simulink model "helicoptertemplate_mp_v2c"  (R2021b)
settings: Solver=ode45  StartTime=0.0  StopTime=Tsim  RelTol=1e-3
InitFcn:
  | hwinit
values from neighbouring files (symbols this model uses):
  A = sysd.A    [MPC_Reference_track.m]    (also in MPC_Reference_track_offset.m; MPC_init_v2.m; MPC_init_v3.m; modelDynamics.m = [0, 1; -(1/J)*g*Mcw*L1*cos(-0.38), -(1/J)*C_alpha])
  B = sysd.B    [MPC_Reference_track.m]    (also in MPC_Reference_track_offset.m; MPC_init_v2.m; MPC_init_v3.m; modelDynamics.m = [0; (1/J)*L2])
  C = sysd.C    [MPC_Reference_track.m]    (also in MPC_Reference_track_offset.m; MPC_init_v2.m; MPC_init_v3.m; modelDynamics.m = [1, 0])
  H = S'*Qbar*S + Rbar    [costgen.m]    (also in costgen_delta.m = S' * Qbar * S + Delta' * Rbar * Delta)
  h = 0.01    [MPC_Reference_track.m]    (also in MPC_Reference_track_offset.m; MPC_init_v2.m; MPC_init_v3.m; costgen.m = [hx0 hxref huref])
  K_i = 1.5    [MPC_init_v2.m]
  sysd = c2d(sys, h)    [MPC_Reference_track.m]    (also in MPC_Reference_track_offset.m; MPC_init_v2.m; MPC_init_v3.m)
  y_ref = -[0.2*ones(1,T_steps/4), 0.3*ones(1,T_steps/4), 0.1*ones(1,T_steps/4), 0.38*ones(1,(T_steps/4)+1),]'    [MPC_Reference_track.m]    (also in MPC_Reference_track_offset.m; MPC_init_v2.m = -0.2; MPC_init_v3.m = -0.1)
undefined symbols (not defined in the file or in its folder): adingain, adinoffs, DiscIntNeverNeededParam, Discrete, h_cost, h_coste, He, HeliMexHandle, LTIe, Time
libraries: ctrlSharedLib x4, eeStairGenerator x2, simulink x1
settings Model: Creator=fkzhang  LastModifiedBy=rjvanderhorst
settings SolverCC: AlgebraicLoopSolver=TrustRegion
settings DataIOCC: LimitDataPoints=on  SaveFormat=Array  ReturnWorkspaceOutputs=off
settings OptimizationCC: BlockReduction=off  BooleanDataType=off  LifeSpan=inf
settings DebuggingCC: AlgebraicLoopMsg=none  SaveWithParameterizedLinksMsg=none  UnderspecifiedInitializationDetection=Classic  MergeDetectMultiDrivingBlocksExec=none  SignalResolutionControl=TryResolveAllWithWarning  AllowSymbolicDim=off  SFUnexpectedBacktrackingDiag=warning  SFNoUnconditionalDefaultTransitionDiag=warning  SFExecutionAtInitializationDiag=none  SFMachineParentedDataDiag=warning  ArithmeticOperatorsInVariantConditions=warning
settings HardwareCC: ProdBitPerPointer=32  ProdBitPerSizeT=32  ProdBitPerPtrDiffT=32  ProdLargestAtomicFloat=None  ProdIntDivRoundTo=Undefined  ProdEndianess=Unspecified  ProdWordSize=32  ProdHWDeviceType=32-bit Generic  TargetUnknown=on
settings ModelReferenceCC: PropagateSignalLabelsOutOfModel=off
settings SFSimCC: SimUseLocalCustomCode=off  CustomCodeUndefinedFunction=UseInterfaceOnly
settings RTWCC: RTWUseLocalCustomCode=off
settings CodeAppCC: StateflowObjectComments=on
settings GRTTargetCC: TargetLangStandard=C89/C90 (ANSI)
settings ConfigComp: CovMetricSettings=dw  CovSaveCumulativeToWorkspaceVar=on  CovSaveSingleToWorkspaceVar=on  CovExternalEMLEnable=off  CovSFcnEnable=off

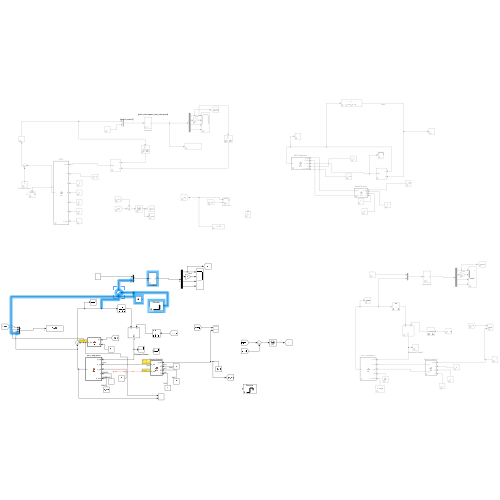
[thumbnail: Simulink's stored preview of the top-level diagram]
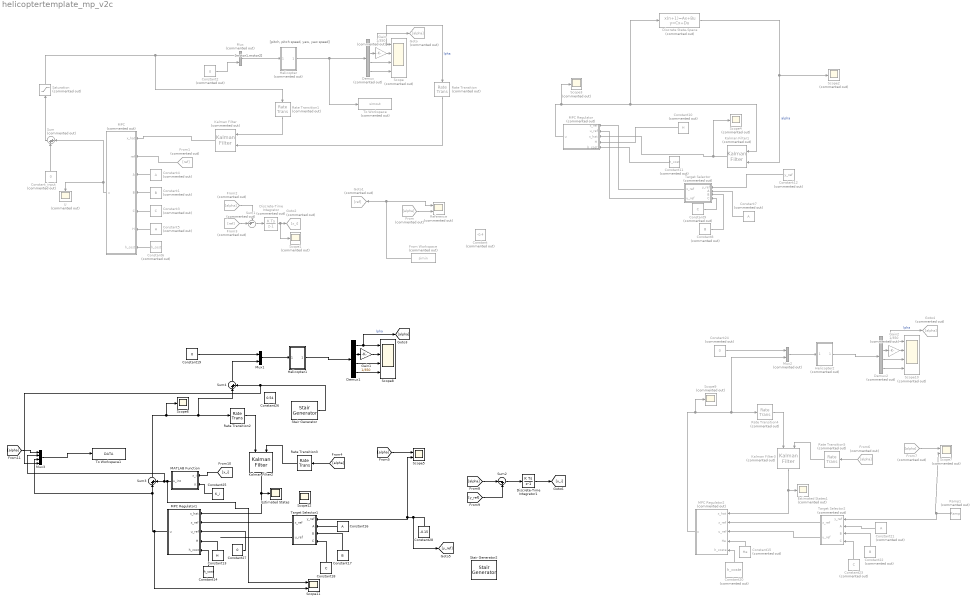
== system helicoptertemplate_mp_v2c ==
  note: [pitch, pitch speed, yaw, yaw speed]
  note: [motor1,motor2]
  " MPC Regulator" : MATLAB Function  Commented=on  TreatAsAtomicUnit=on
  " MPC Regulator1" : MATLAB Function  TreatAsAtomicUnit=on
  " MPC Regulator2" : MATLAB Function  Commented=on  TreatAsAtomicUnit=on
  Constant : Constant  Commented=on  Value=-0.4
  Constant1 : Constant  Commented=on  Value=B  VectorParams1D=off
  Constant10 : Constant  Commented=on  Value=H
  Constant11 : Constant  Commented=on  Value=h_cost
  Constant12 : Constant  Commented=on  Value=y_ref
  Constant13 : Constant  Value=H
  Constant14 : Constant  Value=h_cost
  Constant15 : Constant  Commented=on  Value=He
  Constant16 : Constant  Value=A
  Constant17 : Constant  Value=B  VectorParams1D=off
  Constant18 : Constant  Value=C  VectorParams1D=off
  Constant19 : Constant  Value=0
  Constant2 : Constant  Commented=on  Value=0
  Constant20 : Constant  Commented=on  Value=h_coste
  Constant21 : Constant  Commented=on  Value=A
  Constant22 : Constant  Commented=on  Value=B  VectorParams1D=off
  Constant23 : Constant  Commented=on  Value=C  VectorParams1D=off
  Constant24 : Constant  Commented=on  Value=0
  Constant25 : Constant  Value=K_i
  Constant26 : Constant  Value=0.54  SampleTime=h
  Constant27 : Constant  Value=0
  Constant28 : Constant  Value=-0.15
  Constant3 : Constant  Commented=on  Value=C  VectorParams1D=off
  Constant4 : Constant  Commented=on  Value=A
  Constant5 : Constant  Commented=on  Value=H
  Constant6 : Constant  Commented=on  Value=h_cost
  Constant7 : Constant  Commented=on  Value=A
  Constant8 : Constant  Commented=on  Value=B  VectorParams1D=off
  Constant9 : Constant  Commented=on  Value=C  VectorParams1D=off
  Constant_input : Constant  Commented=on  Value=0
  Demux : Demux  Commented=on
  Demux1 : Demux
  Demux2 : Demux  Commented=on
  Discrete State-Space : DiscreteStateSpace  Commented=on  A=sysd.A  B=sysd.B  C=sysd.C  D=sysd.D  InitialCondition=[0;0]  SampleTime=h
  Discrete-Time Integrator : DiscreteIntegrator  Commented=on  SampleTime=-1  ICPrevOutput=DiscIntNeverNeededParam  ICPrevScaledInput=DiscIntNeverNeededParam
  Discrete-Time Integrator1 : DiscreteIntegrator  SampleTime=h  ICPrevOutput=DiscIntNeverNeededParam  ICPrevScaledInput=DiscIntNeverNeededParam
  Estimated States : Scope
  Estimated States1 : Scope  Commented=on
  From{,2,6..7} (4 alike) : From  Commented=on  GotoTag=alpha
  From Workspace : FromWorkspace  Commented=on  VariableName=simin
  From1 : From  Commented=on  GotoTag=ref
  From3 : From  Commented=on  GotoTag=ref
  Gain : Gain  Commented=on  Gain=1/350
  Gain1 : Gain  Gain=1/350
  Gain2 : Gain  Commented=on  Gain=1/350
  Goto : Goto  Commented=on  GotoTag=alpha
  Goto1 : Goto  Commented=on  GotoTag=ref
  Goto2 : Goto  Commented=on  GotoTag=x_i
  Goto4 : Goto  Commented=on  GotoTag=alpha
  Helicopter : Subsystem  Commented=on  mask{Ts=h}
      mask prompts: Ts "sampletime"
      mask init:
      | sf_heli_init
      mask Display:
      | port_label('input',1,'u');
      | port_label('output',1,'y');
  Helicopter1 : Subsystem  mask{Ts=h}
      mask prompts: Ts "sampletime"
      mask init:
      | sf_heli_init
      mask Display:
      | port_label('input',1,'u');
      | port_label('output',1,'y');
  Helicopter2 : Subsystem  Commented=on  mask{Ts=h}
      mask prompts: Ts "sampletime"
      mask init:
      | sf_heli_init
      mask Display:
      | port_label('input',1,'u');
      | port_label('output',1,'y');
  Kalman Filter : ctrlSharedLib/Kalman Filter  Commented=on  TimeDomain=Discrete-Time  UseCurrentEstimator=on  ModelSource=Individual A, B, C, D matrices  ModelSourceVariable=ss(0.95,1,1,0,1)  A=sysd.A  B=sysd.B  C=sysd.C  D=sysd.D  NumberOfStates=1  NumberOfInputs=1  NumberOfOutputs=1  InitialEstimateSource=Dialog  X0=[0; 0]  P0=10  UseK=off  UseGH=off  NumberOfProcessNoiseInputs=1  G=1  TimeInvariantG=on  H=0  TimeInvariantH=on  Q=0.05  TimeInvariantQ=on  R=1  TimeInvariantR=on  N=0  TimeInvariantN=on  AddInputPort=on  AddEnablePort=off  OutputEstimatedY=off  OutputP=off  Ts=h
  Kalman Filter1 : ctrlSharedLib/Kalman Filter  Commented=on  TimeDomain=Discrete-Time  UseCurrentEstimator=on  ModelSource=Individual A, B, C, D matrices  ModelSourceVariable=ss(0.95,1,1,0,1)  A=sysd.A  B=sysd.B  C=sysd.C  D=sysd.D  NumberOfStates=1  NumberOfInputs=1  NumberOfOutputs=1  InitialEstimateSource=Dialog  X0=[0; 0]  P0=10  UseK=off  UseGH=off  NumberOfProcessNoiseInputs=1  G=1  TimeInvariantG=on  H=0  TimeInvariantH=on  Q=0.05  TimeInvariantQ=on  R=1  TimeInvariantR=on  N=0  TimeInvariantN=on  AddInputPort=on  AddEnablePort=off  OutputEstimatedY=off  OutputP=off  Ts=-1
  Kalman Filter2 : ctrlSharedLib/Kalman Filter  TimeDomain=Discrete-Time  UseCurrentEstimator=on  ModelSource=Individual A, B, C, D matrices  ModelSourceVariable=ss(0.95,1,1,0,1)  A=sysd.A  B=sysd.B  C=sysd.C  D=sysd.D  NumberOfStates=1  NumberOfInputs=1  NumberOfOutputs=1  InitialEstimateSource=Dialog  X0=[0; 0]  P0=10  UseK=off  UseGH=off  NumberOfProcessNoiseInputs=1  G=1  TimeInvariantG=on  H=0  TimeInvariantH=on  Q=0.05  TimeInvariantQ=on  R=1  TimeInvariantR=on  N=0  TimeInvariantN=on  AddInputPort=on  AddEnablePort=off  OutputEstimatedY=off  OutputP=off  Ts=-1
  Kalman Filter3 : ctrlSharedLib/Kalman Filter  Commented=on  TimeDomain=Discrete-Time  UseCurrentEstimator=on  ModelSource=Individual A, B, C, D matrices  ModelSourceVariable=ss(0.95,1,1,0,1)  A=LTIe.A  B=LTIe.B  C=LTIe.C  D=0  NumberOfStates=1  NumberOfInputs=1  NumberOfOutputs=1  InitialEstimateSource=Dialog  X0=[0; 0; 0]  P0=10  UseK=off  UseGH=off  NumberOfProcessNoiseInputs=1  G=1  TimeInvariantG=on  H=0  TimeInvariantH=on  Q=0.05  TimeInvariantQ=on  R=1  TimeInvariantR=on  N=0  TimeInvariantN=on  AddInputPort=on  AddEnablePort=off  OutputEstimatedY=off  OutputP=off  Ts=-1
  MATLAB Function : MATLAB Function  TreatAsAtomicUnit=on
  MPC : MATLAB Function  Commented=on  TreatAsAtomicUnit=on
  Mux : Mux  Commented=on  Inputs=2
  Mux1 : Mux  Inputs=2
  Mux2 : Mux  Commented=on  Inputs=2
  Mux3 : Mux
  Ramp1 : simulink/Sources/Ramp  Commented=on  slope=0  start=0  InitialOutput=-0.15
  Rate Transition{,1,4..5} (4 alike) : RateTransition  Commented=on  OutPortSampleTime=h
  Rate Transition2 : RateTransition  OutPortSampleTime=h
  Rate Transition3 : RateTransition  OutPortSampleTime=h
  Reference : Scope  Commented=on  NumInputPorts=2
  Saturation : Saturate  Commented=on  UpperLimit=1  LowerLimit=-1
  Scope : Scope  Commented=on  NumInputPorts=4
  Scope{1..4,9} (5 alike) : Scope  Commented=on
  Scope10 : Scope  Commented=on  NumInputPorts=4
  Scope11 : Scope  NumInputPorts=2
  Scope12 : Scope
  Scope5 : Scope  NumInputPorts=2
  Scope6 : Scope
  Scope7 : Scope  Commented=on  NumInputPorts=2
  Scope8 : Scope  NumInputPorts=4
  Stair Generator : eeStairGenerator/Stair Generator  LabelModeActiveChoice=Discrete  TimeInput=[0 20 21 ]  AmplitudeInput=[0 1 0]  SampleTime=h  RepeatPattern=off  OutDataTypeStr=double
      settings: SourceProductBaseCode=PS
  Stair Generator2 : eeStairGenerator/Stair Generator  LabelModeActiveChoice=Discrete  TimeInput=[0 20 40]  AmplitudeInput=[-0.15 -0.05 -0.1]  SampleTime=h  RepeatPattern=off  OutDataTypeStr=double
      settings: SourceProductBaseCode=PS
  Sum : Sum  Commented=on  Inputs=|++
  Sum1 : Sum  Commented=on  Inputs=-+|
  Sum2 : Sum  Inputs=|-+
  Sum3 : Sum  Inputs=|++
  Sum4 : Sum  Inputs=|++
  Target Selector : MATLAB Function  Commented=on  TreatAsAtomicUnit=on
  Target Selector1 : MATLAB Function  TreatAsAtomicUnit=on
  Target Selector2 : MATLAB Function  Commented=on  TreatAsAtomicUnit=on
  To Workspace : ToWorkspace  Commented=on  VariableName=simout  SaveFormat=Structure With Time  SampleTime=-1
  To Workspace1 : ToWorkspace  VariableName=DATA  SaveFormat=Timeseries  SampleTime=h
  U : Scope  Commented=on
  wires:
  Helicopter/1(Out1) -> To Workspace/1, Demux/1
  Mux/1 -> Helicopter/1(In1)
  Constant2/1 -> Mux/2
  Demux/3 -> Scope/3
  Demux/4 -> Scope/4
  Demux/2 -> Gain/1
  Gain/1 -> Scope/2
  Demux/1 -> Goto/1, Rate Transition/1, Scope/1  "lpha"
  Constant_input/1 -> Sum/2
  Sum/1 -> Saturation/1
  MPC/1(u) -> Sum/1, U/1
  Kalman Filter/1 -> MPC/1(x_hat)
  Saturation/1 -> Rate Transition1/1, Mux/1
  Rate Transition/1 -> Kalman Filter/2
  From/1 -> Reference/2
  From Workspace/1 -> Reference/1, Goto1/1
  From2/1 -> Sum1/1
  From3/1 -> Sum1/2
  Sum1/1 -> Discrete-Time Integrator/1
  Discrete-Time Integrator/1 -> Scope1/1, Goto2/1
  Constant1/1 -> MPC/4(B)
  Constant3/1 -> MPC/5(C)
  Constant4/1 -> MPC/3(A)
  Constant5/1 -> MPC/6(H)
  Constant6/1 -> MPC/7(h_cost)
  Rate Transition1/1 -> Kalman Filter/1
  From1/1 -> MPC/2(ref)
  Discrete State-Space/1 -> Scope2/1, Kalman Filter1/2  "alpha"
  " MPC Regulator"/1(u) -> Scope3/1, Kalman Filter1/1, Discrete State-Space/1
  Kalman Filter1/1 -> Scope4/1, " MPC Regulator"/3(x_hat)
  Target Selector/1(x_ref) -> " MPC Regulator"/1(x_ref)
  Target Selector/2(u_ref) -> " MPC Regulator"/2(u_ref)
  Constant7/1 -> Target Selector/2(A)
  Constant9/1 -> Target Selector/4(C)
  Constant8/1 -> Target Selector/3(B)
  Constant11/1 -> " MPC Regulator"/5(h_cost)
  Constant10/1 -> " MPC Regulator"/4(H)
  Constant12/1 -> Target Selector/1(y_ref)
  Constant18/1 -> Target Selector1/4(C)
  Target Selector1/1(x_ref) -> " MPC Regulator1"/2(x_ref)
  Constant14/1 -> " MPC Regulator1"/5(h_cost)
  Constant13/1 -> " MPC Regulator1"/4(H)
  Constant17/1 -> Target Selector1/3(B)
  Constant16/1 -> Target Selector1/2(A)
  Constant28/1 -> [y_ref], Target Selector1/1(y_ref), Scope5/2
  Kalman Filter2/1 -> Estimated States/1, " MPC Regulator1"/1(x_hat)
  Constant19/1 -> Mux1/1
  Mux1/1 -> Helicopter1/1(In1)
  Demux1/2 -> Gain1/1
  Demux1/4 -> Scope8/4
  Gain1/1 -> Scope8/2
  Helicopter1/1(Out1) -> Demux1/1
  Demux1/1 -> [alpha], Scope8/1  "lpha"
  Demux1/3 -> Scope8/3
  Rate Transition2/1 -> Kalman Filter2/1
  [alpha] -> Rate Transition3/1
  Rate Transition3/1 -> Kalman Filter2/2
  [alpha] -> Scope5/1
  Demux2/3 -> Scope10/3
  Gain2/1 -> Scope10/2
  Demux2/4 -> Scope10/4
  Demux2/1 -> Goto4/1, Scope10/1  "lpha"
  Kalman Filter3/1 -> Estimated States1/1, " MPC Regulator2"/1(x_hat)
  Constant22/1 -> Target Selector2/3(B)
  Helicopter2/1(Out1) -> Demux2/1
  Constant21/1 -> Target Selector2/2(A)
  Constant15/1 -> " MPC Regulator2"/4(He)
  Constant20/1 -> " MPC Regulator2"/5(h_coste)
  Target Selector2/1(x_ref) -> " MPC Regulator2"/2(x_ref)
  Constant23/1 -> Target Selector2/4(C)
  Mux2/1 -> Helicopter2/1(In1)
  Demux2/2 -> Gain2/1
  Rate Transition4/1 -> Kalman Filter3/1
  Ramp1/1 -> Target Selector2/1(y_ref), Scope7/2
  From6/1 -> Rate Transition5/1
  Rate Transition5/1 -> Kalman Filter3/2
  Constant24/1 -> Mux2/1
  From7/1 -> Scope7/1
  Target Selector2/2(u_ref) -> " MPC Regulator2"/3(u_ref)
  " MPC Regulator2"/1(u) -> Scope9/1, Mux2/2, Rate Transition4/1
  [alpha] -> Sum2/1
  [y_ref] -> Sum2/2
  Sum2/1 -> Discrete-Time Integrator1/1
  Discrete-Time Integrator1/1 -> [x_i]
  [x_i] -> MATLAB Function/1(x_i)
  Constant25/1 -> MATLAB Function/2(K)
  " MPC Regulator1"/1(u) -> Mux3/3, Sum3/1, Scope11/2
  Sum4/1 -> Mux1/2
  MATLAB Function/1(u_int) -> Scope11/1, Mux3/2, Sum3/2
  Target Selector1/2(u_ref) -> ?
  Constant27/1 -> " MPC Regulator1"/3(u_ref)
  Sum3/1 -> Scope6/1, Sum4/1, Rate Transition2/1
  Mux3/1 -> To Workspace1/1
  [alpha] -> Mux3/1
  Stair Generator/1 -> Mux3/4, Sum4/2

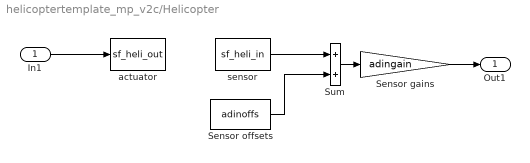
== system helicoptertemplate_mp_v2c/Helicopter ==
  In1 : Inport
  Sensor gains : Gain  Gain=adingain
  Sensor offsets : Constant  Value=adinoffs
  Sum : Sum
  actuator : M-S-Function  FunctionName=sf_heli_out  Parameters=HeliMexHandle,Ts
  sensor : M-S-Function  FunctionName=sf_heli_in  Parameters=HeliMexHandle
  Out1 : Outport
  wires:
  sensor/1 -> Sum/1
  In1/1 -> actuator/1
  Sensor offsets/1 -> Sum/2
  Sum/1 -> Sensor gains/1
  Sensor gains/1 -> Out1/1

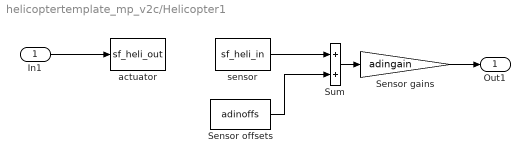
== system helicoptertemplate_mp_v2c/Helicopter1 ==
  In1 : Inport
  Sensor gains : Gain  Gain=adingain
  Sensor offsets : Constant  Value=adinoffs
  Sum : Sum
  actuator : M-S-Function  FunctionName=sf_heli_out  Parameters=HeliMexHandle,Ts
  sensor : M-S-Function  FunctionName=sf_heli_in  Parameters=HeliMexHandle
  Out1 : Outport
  wires:
  sensor/1 -> Sum/1
  In1/1 -> actuator/1
  Sensor offsets/1 -> Sum/2
  Sum/1 -> Sensor gains/1
  Sensor gains/1 -> Out1/1

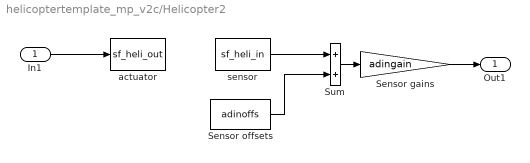
== system helicoptertemplate_mp_v2c/Helicopter2 ==
  In1 : Inport
  Sensor gains : Gain  Gain=adingain
  Sensor offsets : Constant  Value=adinoffs
  Sum : Sum
  actuator : M-S-Function  FunctionName=sf_heli_out  Parameters=HeliMexHandle,Ts
  sensor : M-S-Function  FunctionName=sf_heli_in  Parameters=HeliMexHandle
  Out1 : Outport
  wires:
  sensor/1 -> Sum/1
  In1/1 -> actuator/1
  Sensor offsets/1 -> Sum/2
  Sum/1 -> Sensor gains/1
  Sensor gains/1 -> Out1/1

== matlab function helicoptertemplate_mp_v2c/ MPC Regulator ==
  data: x_ref input; u output; u_ref input; x_hat input; H input; h_cost input
function u = fcn(x_ref, u_ref, x_hat, H, h_cost)
    u = zeros(1,1);
    x_0=x_hat;
    
    N = 10;
    
    coder.extrinsic('quadprog');
    % options = optimoptions(@quadprog);
    
    lb = -1*ones(N, 1);
    ub = -1*lb;
    
    uN = quadprog(H,(h_cost*[x_0; x_ref; u_ref]),[],[],[],[],lb,ub,[]);

    % Select the first input only
    u=uN(1);
    
end

== matlab function helicoptertemplate_mp_v2c/MPC ==
  data: x_hat input; ref input; A input; B input; u output; C input; H input; h_cost input
function u = fcn(x_hat, ref, A, B, C, H, h_cost)
      
    u = zeros(1,1); % Define the output type for the extrinsic call.
    
    N = 20; %prediction horizon
    coder.extrinsic('quadprog');
    A_OT = [eye(2)-A, -B; C, zeros(1,1)];
    disp(size(A_OT))
    B_OT = [zeros(2,1); ref];
    
    H_ots = [0 0 0;
             0 0 0;
             0 0 1];
    
    lb_ots = [-10000; 0; -1];
    ub_ots = -lb_ots;
    
    %options = optimoptions('fmincon', 'Algorithm','sqp');
    OTS = quadprog(H_ots,[],[],[],A_OT,B_OT,lb_ots,ub_ots,[]);
    x_ref = OTS(1:2);
    u_ref = OTS(3);
    %%%%%%%%%%%%%%%%%%%%%%%%%%%OTS%%%%%%%%%%%%%%%%%%%%%%%%%%%%


    

    %%%%%%%%%%%%%%%%%%%%%%%%%%%MPC%%%%%%%%%%%%%%%%%%%%%%%%%%%%
    x_0=x_hat;
    
    lb = -1*ones(N,1);
    ub = -0*lb;
    uN = quadprog(H,(h_cost*[x_0; x_ref; u_ref]),[],[],[],[],lb,ub,[]);

    % Select the first input only
    u=uN(1);

end

== matlab function helicoptertemplate_mp_v2c/Target Selector ==
  data: y_ref input; x_ref output; u_ref output; A input; B input; C input
function [x_ref, u_ref] = fcn(y_ref, A, B, C)
    x_ref = [0; 0];
    u_ref = 0;
    coder.extrinsic('quadprog');
    A_OT = [eye(2)-A, -B; C, 0];
    B_OT = [zeros(2,1); y_ref];
    
    H_ots = [0 0 0;
             0 0 0;
             0 0 1];
    
    lb_ots = [-10000; 0; -1];
    ub_ots = -lb_ots;
    
    % options = optimoptions(@quadprog);
    OTS = quadprog(H_ots,[],[],[],A_OT,B_OT,lb_ots,ub_ots,[]);
    x_ref = OTS(1:2);
    u_ref = OTS(3);
end

== matlab function helicoptertemplate_mp_v2c/ MPC Regulator1 ==
  data: x_hat input; x_ref input; u output; u_ref input; H input; h_cost input
function u = fcn(x_hat, x_ref, u_ref, H, h_cost)
    u = zeros(1,1);
    x_0=x_hat;
    
    N = 20;
    
    coder.extrinsic('quadprog');
    coder.extrinsic('warning');
    % options = optimoptions(@quadprog);
    warning('off','all');
    
    ub = 1.5*ones(N, 1);
    lb = 0*ub;
    options = optimset('Display','off');
    uN = quadprog(H,(h_cost*[x_0; x_ref; u_ref]),[],[],[],[],lb,ub,[],options);
    warning('on','all');
    % Select the first input only
    u=uN(1);
    
end

== matlab function helicoptertemplate_mp_v2c/Target Selector1 ==
  data: y_ref input; x_ref output; u_ref output; A input; B input; C input
function [x_ref, u_ref] = fcn(y_ref, A, B, C)
    x_ref = [0; 0];
    u_ref = 0;
    coder.extrinsic('quadprog');
    A_OT = [eye(2)-A, -B; C, 0];
    B_OT = [zeros(2,1); y_ref];
    
    H_ots = [0 0 0;
             0 0 0;
             0 0 1];
    
    lb_ots = [-10000; 0; -1];
    ub_ots = -lb_ots;
    
    % options = optimoptions(@quadprog);
    options = optimset('Display','off');
    OTS = quadprog(H_ots,[],[],[],A_OT,B_OT,lb_ots,ub_ots,[],options);
    x_ref = OTS(1:2);
    u_ref = OTS(3);
end

== matlab function helicoptertemplate_mp_v2c/ MPC Regulator2 ==
  data: x_hat input; x_ref input; u output; u_ref input; He input; h_coste input
function u = fcn(x_hat, x_ref, u_ref, He, h_coste)
    u = zeros(1,1);
    x_0=x_hat;

    xre = [x_ref; x_hat(3)];
    
    N = 100;
    
    coder.extrinsic('quadprog');
    % options = optimoptions(@quadprog);
    
    ub = ones(N, 1);
    lb = 0*ub;
    
    uN = quadprog(He,(h_coste*[x_0; xre; u_ref]),[],[],[],[],lb,ub,[]);

    % Select the first input only
    u=uN(1);
    
end

== matlab function helicoptertemplate_mp_v2c/Target Selector2 ==
  data: y_ref input; x_ref output; u_ref output; A input; B input; C input
function [x_ref, u_ref] = fcn(y_ref, A, B, C)
    x_ref = [0; 0];
    u_ref = 0;
    coder.extrinsic('quadprog');
    A_OT = [eye(2)-A, -B; C, 0];
    B_OT = [zeros(2,1); y_ref];
    
    H_ots = [0 0 0;
             0 0 0;
             0 0 1];
    
    lb_ots = [-10000; 0; -1];
    ub_ots = -lb_ots;
    
    % options = optimoptions(@quadprog);
    OTS = quadprog(H_ots,[],[],[],A_OT,B_OT,lb_ots,ub_ots,[]);
    x_ref = OTS(1:2);
    u_ref = OTS(3);
end

== matlab function helicoptertemplate_mp_v2c/MATLAB Function ==
  data: x_i input; u_int output; K input
function u_int = fcn(x_i, K)
    u_int = -K*x_i;
